simulink model "Ring_modulator"  (Simulink 10.0)
settings: Solver=ode45  StartTime=0.0  StopTime=0.001  MaxStep=2e-6  RelTol=1e-15  AbsTol=1e-18  EnableMultiTasking=on
settings Model: Creator=UX31  LastModifiedBy=unknown
settings SolverCC: AutoScaleAbsTol=off  ZeroCrossAlgorithm=Adaptive
settings DataIOCC: LimitDataPoints=on
settings DebuggingCC: UnderspecifiedInitializationDetection=Simplified  MergeDetectMultiDrivingBlocksExec=error  TimeAdjustmentMsg=warning  SolverPrmCheckMsg=warning
settings GRTTargetCC: GeneratePreprocessorConditionals=Disable all  CombineOutputUpdateFcns=on  GRTInterface=off
settings ConfigComp: CovExternalEMLEnable=off  CovSFcnEnable=off

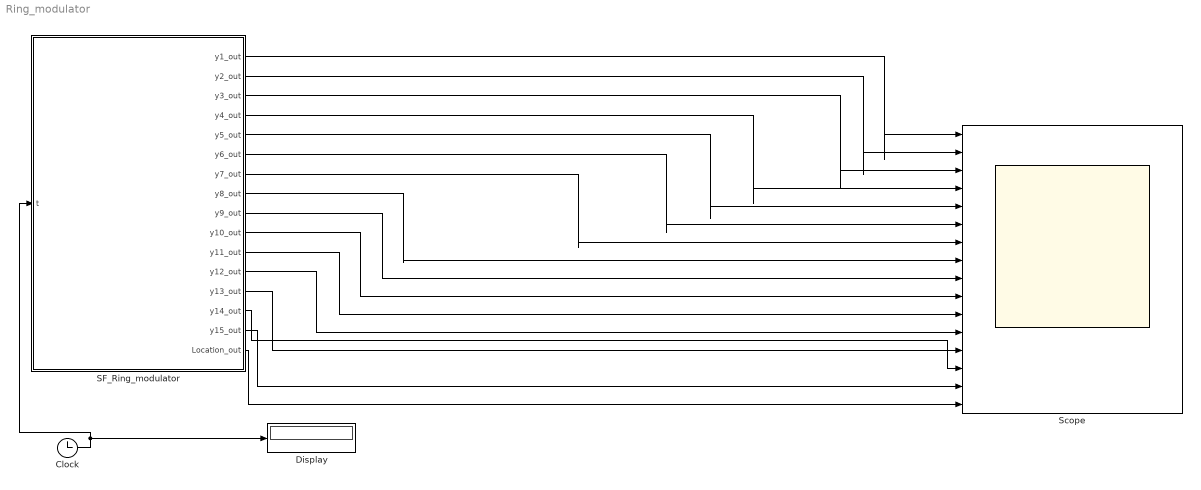
== system Ring_modulator ==
  Clock : Clock
  Display : Display
  SF_Ring_modulator : Stateflow chart  TreatAsAtomicUnit=on
  Scope : Scope  NumInputPorts=16
  wires:
  SF_Ring_modulator/1(y1_out) -> Scope/1
  SF_Ring_modulator/2(y2_out) -> Scope/2
  SF_Ring_modulator/3(y3_out) -> Scope/3
  SF_Ring_modulator/4(y4_out) -> Scope/4
  SF_Ring_modulator/5(y5_out) -> Scope/5
  SF_Ring_modulator/6(y6_out) -> Scope/6
  SF_Ring_modulator/7(y7_out) -> Scope/7
  SF_Ring_modulator/8(y8_out) -> Scope/8
  SF_Ring_modulator/9(y9_out) -> Scope/9
  SF_Ring_modulator/10(y10_out) -> Scope/10
  SF_Ring_modulator/11(y11_out) -> Scope/11
  SF_Ring_modulator/12(y12_out) -> Scope/12
  SF_Ring_modulator/13(y13_out) -> Scope/13
  SF_Ring_modulator/14(y14_out) -> Scope/14
  SF_Ring_modulator/15(y15_out) -> Scope/15
  SF_Ring_modulator/16(Location_out) -> Scope/16
  Clock/1 -> Display/1, SF_Ring_modulator/1(t)

== stateflow chart SF_Ring_modulator ==
  settings: updateMethod=CONTINUOUS
  state Ring_modulator
    du:
    y1_dot=(C^-1)*(y8-0.5*y10+0.5*y11+y14-(R^-1)*y1);
    y2_dot=(C^-1)*(y9-0.5*y12+0.5*y13+y15-(R^-1)*y2);
    y3_dot=(Cs^-1)*(y10 - gamma*(exp(theta*(y3-y5-y7-2*sin(20000*pi*t)))-1) + gamma*(exp(theta*(-y3-y6+y7+ 2*sin(20000*pi*t)))-1));
    y4_dot=(Cs^-1)*(-y11+ gamma*(exp(theta*(-y4+y6-y7-2*sin(20000*pi*t)))-1) + gamma*(exp(theta*(y4+y5+y7+2*sin(20000*pi*t)))-1));
    y5_dot=(Cs^-1)*(y12+ gamma*(exp(theta*(y3-y5-y7-2*sin(20000*pi*t)))-1) - gamma*(exp(theta*(y4+y5+y7+2*sin(20000*pi*t)))-1));
    y6_dot=(Cs^-1)*(-y13 - gamma*(exp(theta*(-y4+y6-y7-2*sin(20000*pi*t)))-1) + gamma*(exp(theta*(-y3-y6+y7+ 2*sin(20000*pi*t)))-1));
    y7_dot=(Cp^-1)*(-(Rp^-1)*y7 + gamma*(exp(theta*(y3-y5-y7-2*sin(20000*pi*t)))-1) + gamma*(exp(theta*(-y4+y6-y7-2*sin(20000*pi*t)))-1) - gamma*(exp(theta*(y4+y5+y7+2*sin(20000*pi*t)))-1) - gamma*(exp(theta*(-y3-y6+y7+ 2*sin(20000*pi*t)))-1));
    y8_dot=-(Lh^-1)*y1;
    y9_dot=-(Lh^-1)*y2;
    y10_dot=(Ls2^-1)*(0.5*y1-y3-Rg2*y10);
    y11_dot=(Ls3^-1)*(-0.5*y1+y4-Rg3*y11);
    y12_dot=(Ls2^-1)*(0.5*y2-y5-Rg2*y12);
    y13_dot=(Ls3^-1)*(-0.5*y2+y6-Rg3*y13);
    y14_dot=(Ls1^-1)*(-y1 + 0.5*sin(2000*pi*t));
    y15_dot=(Ls1^-1)*(-y2-(Rc+Rg1)*y15);
    y1_out=y1;
    y2_out=y2;
    y3_out=y3;
    y4_out=y4;
    y5_out=y5;
    y6_out=y6;
    y7_out=y7;
    y8_out=y8;
    y9_out=y9;
    y10_out=y10;
    y11_out=y11;
    y12_out=y12;
    y13_out=y13;
    y14_out=y14;
    y15_out=y15;
    Location_out =1;
  (default) -> Ring_modulator : {y1=0;y2=0;y3=0;y4=0;y5=0;y6=0;y7=0;y8=0;y9=0;y10=0;y11=0;y12=0;y13=0;y14=0;y15=0}
  data: y1 local double; y1_out output double; y2 local double; y2_out output double; y3 local double; y3_out output double; y4 local double; y4_out output double; y5 local double; y5_out output double; y6 local double; y6_out output double; y7 local double; y7_out output double; y8 local double; y8_out output double; y9 local double; y9_out output double; y10 local double; y10_out output double; y11 local double; y11_out output double; y12 local double; y12_out output double; y13 local double; y13_out output double; y14 local double; y14_out output double; y15 local double; y15_out output double; Location_out output double; C constant double =1.6*10^-8; Cs constant double =2*10^-12; Cp constant double =10^-8; Lh constant double =4.45; Ls1 constant double =0.002; Ls2 constant double =5*10^-4; Ls3 constant double =5*10^-4; gamma constant double =40.67286402*10^-9; R constant double =25000; Rp constant double =50; Rg1 constant double =36.3; Rg2 constant double =17.3; Rg3 constant double =17.3; Ri constant double =50; Rc constant double =600; theta constant double =17.7493332; pi constant double =3.1415926535; t input double
  data y1 settings: updateMethod=SF_CONTINUOUS_TIME_DATA
  data y2 settings: updateMethod=SF_CONTINUOUS_TIME_DATA
  data y3 settings: updateMethod=SF_CONTINUOUS_TIME_DATA
  data y4 settings: updateMethod=SF_CONTINUOUS_TIME_DATA
  data y5 settings: updateMethod=SF_CONTINUOUS_TIME_DATA
  data y6 settings: updateMethod=SF_CONTINUOUS_TIME_DATA
  data y7 settings: updateMethod=SF_CONTINUOUS_TIME_DATA
  data y8 settings: updateMethod=SF_CONTINUOUS_TIME_DATA
  data y9 settings: updateMethod=SF_CONTINUOUS_TIME_DATA
  data y10 settings: updateMethod=SF_CONTINUOUS_TIME_DATA
  data y11 settings: updateMethod=SF_CONTINUOUS_TIME_DATA
  data y12 settings: updateMethod=SF_CONTINUOUS_TIME_DATA
  data y13 settings: updateMethod=SF_CONTINUOUS_TIME_DATA
  data y14 settings: updateMethod=SF_CONTINUOUS_TIME_DATA
  data y15 settings: updateMethod=SF_CONTINUOUS_TIME_DATA
